simulink model "dvbs2_stream"  (R2024b)
settings: Solver=FixedStepDiscrete  StartTime=0.0  StopTime=18000/Fs  RelTol=1e-3
PreLoadFcn:
  | Rs = 125e3;
  | Fs = 8*Rs;
  | nsamp = 4096;
  | t = (0:nsamp)/Fs;
  | y = randi(2^8-1,1,2048);
  | ly = length(y);
InitFcn:
  | Rs = 125e3;
  | Fs = 8*Rs;
  | nsamp = 4096;
  | t = (0:nsamp)/Fs;
  | y = randi(2^8-1,1,2048);
  | ly = length(y);
libraries: hdlsllib x132, simulink x41, dspsigops x7, commseqgen3 x5, whdlutilities x5, commhdlcrc x2, dsphdlfiltering2 x1, whdlmod x1, sdrzblksprivate x1
(part 6 of 6)

== matlab function dvbs2_stream/HDL_DUT/Tx/DVB-S2 Tx/FEC Encoder/DVB-S2 LDPC Encoder/ParityController ==
  data: ird_addr output; pwr_addr output; pwr_enb output; prd_addr output; endEnc input; paraddr input; encenable input; inpLen input; parLen input; qfactor input; noofcol input; reset input; starto output; endo output; valido output; par_ind output; i_index output; p_index output; framevalid input
function [ird_addr,pwr_addr,pwr_enb,prd_addr,starto,endo,valido,par_ind,...
    i_index,p_index] = ParityController(endEnc,paraddr,encenable,...
    inpLen,parLen,qfactor,noofcol,reset,framevalid)

persistent validO prdAddr pwrAddr pwrEnb pwrEnbReg ...
    irdAddr prdEnb endValid startO icountZ inCount ...
    parCount pcountZ;
if isempty(validO)
    validO = false;
    prdAddr = uint8(1);
    pwrAddr = uint8(0);
    irdAddr = uint8(1);
    pwrEnb = false;
    pwrEnbReg = false;
    prdEnb = false;
    endValid = false;
    startO = false;
    icountZ = fi(1,0,9,0,hdlfimath);
    pcountZ = fi(1,0,9,0,hdlfimath);
    inCount = fi(0,0,16,0,hdlfimath);
    parCount = fi(0,0,16,0,hdlfimath);
end

ird_addr = irdAddr;
pwr_addr = pwrAddr;
prd_addr = prdAddr;
pwr_enb =  pwrEnbReg;
starto = startO;
par_ind = prdEnb;

i_index = icountZ;
p_index = pcountZ;

% Control signals
startO = endEnc;
endo = endValid;
valido = validO && ~endValid;

pwrEnbReg(:) = pwrEnb;

if reset
    prdAddr(:) = 1;
    pwrAddr(:) = 0;
    pwrEnb(:) = false;
    prdEnb(:) = false;
    endValid(:) = false;
    irdAddr(:) = 1;
    icountZ(:) = 1;
    pcountZ(:) = 1;
    inCount(:) = 0;
    parCount(:) = 0;
else
    if validO
        pwrEnb(:) = false;
        pwrAddr(:) = 0;

        if ~prdEnb
            if icountZ == fi(360,0,9,0,hdlfimath)
                if ~(irdAddr == noofcol)
                    irdAddr(:) = irdAddr + 1;
                end
                icountZ(:) = 1;
            else
                icountZ(:) = icountZ + 1;
            end
        end

        if inCount == inpLen
            prdEnb(:) = true;
        else
            inCount(:) = inCount + 1;
        end

        if prdEnb
            if parCount == parLen
                prdEnb(:) = false;
                endValid(:) = true;
            else
                parCount(:) = parCount + 1;
                if prdAddr == fi(qfactor,0,9,0,hdlfimath)
                    prdAddr(:) = 1;
                    if pcountZ == fi(360,0,9,0,hdlfimath)
                        pcountZ(:) = 1;
                    else
                        pcountZ(:) = pcountZ + 1;
                    end
                else
                    prdAddr(:) = prdAddr + 1;
                end
            end
        else
            prdAddr(:) = 1;
            endValid(:) = false;
        end
    else
        if framevalid
            pwrEnb(:) = true;
            if pwrAddr == uint8(255)
                pwrAddr(:) = 1;
            else
                pwrAddr(:) = pwrAddr+1;
            end
        else
            if encenable
                pwrEnb(:) = true;
            else
                pwrEnb(:) = false;
            end
            pwrAddr(:) = prdAddr;
        end
        prdAddr(:) = paraddr;
        prdEnb(:) = false;
        endValid(:) = false;
    end
end

if reset || endValid
    validO(:) = false;
elseif endEnc
    validO(:) = true;
end

== matlab function dvbs2_stream/HDL_DUT/Tx/DVB-S2 Tx/FEC Encoder/DVB-S2 LDPC Encoder/inputController ==
  data: reset output; datai input; iwr_data output size=360; iwr_addr output; starti input; endi input; validi input; fecframe input; coderate input; iwr_enb output size=360; ird_addr output; encenable output; addridx output; rdenable input; encend input; framevalid output; noofcol input
function [reset,iwr_data, iwr_addr,iwr_enb,ird_addr,encenable,addridx,framevalid] = ...
    inputController(datai,starti,endi,validi,fecframe,coderate,rdenable,encend,noofcol)
%#codegen

persistent fecFrame codeRate dataReg endReg validReg frameValid  frameValidReg...
           iwrData iwrAddr iwrEnb irdAddr idxCount wrCount encEnb disValid;
if isempty(dataReg)
    fecFrame = fi(0,0,1,0);
    codeRate = fi(0,0,4,0);
    dataReg = cast(0,'like',datai);
    endReg = false;
    validReg = false;
    frameValid = false;
    frameValidReg = false;
    iwrData = cast(zeros(360,1),'like',datai);
    iwrAddr = fi(0,0,8,0,hdlfimath);
    iwrEnb  = zeros(360,1)>0;
    irdAddr = fi(0,0,8,0,hdlfimath);
    idxCount = fi(1,0,9,0,hdlfimath);
    wrCount = fi(1,0,8,0,hdlfimath);
    encEnb = false;
    disValid = false;
end

% outputs
iwr_data = iwrData;
iwr_addr = iwrAddr;
iwr_enb = iwrEnb;
ird_addr = irdAddr;
encenable = disValid;

%% reset signal
reset = starti && validi;

%% Sample fecFrame and codeRate - Calculate input,parity length and address index.
if reset
    fecFrame(:) = fecframe;
    codeRate(:) = coderate;
end

addridx = fi(bitconcat(fecFrame,codeRate),0,5,0);

%% Reading data
if reset
    irdAddr(:) = 1;
else
    if rdenable
        if irdAddr == cast(noofcol,'like',irdAddr)
            irdAddr(:) = 1;
        else
            irdAddr(:) = irdAddr + 1;
        end
    end
end

%% Writing and Reading data into Input Bits RAM
if reset
    iwrData(:) = zeros(360,1);
    iwrAddr(:) = 0;
    iwrEnb(:) = zeros(360,1);
    idxCount(:) = 1;
    wrCount(:) = 1;
else
    if frameValid && validReg
        for idx = 1:360
            if idxCount == fi(idx,0,9,0)
                iwrEnb(idx) = true;
                iwrData(idx) = dataReg;
            else
                iwrEnb(idx) = false;
                iwrData(idx) = 0;
            end
        end
        iwrAddr(:) = wrCount;
        if idxCount == fi(360,0,9,0)
            idxCount(:) = 1;
            wrCount(:) = wrCount + 1;
        else
            idxCount(:) = idxCount + 1;
        end
    else
        iwrData(:) = 0;
        iwrEnb(:)  = false;
    end
end

if reset
    frameValid(:) = true;
    encEnb(:) = false;
elseif endReg && validReg
    frameValid(:) = false;
    encEnb(:) = true;
elseif encend
    encEnb(:) = false;
end

if reset
    frameValidReg(:) = true;
elseif endi && validi
    frameValidReg(:) = false;
end

if encEnb
    disValid(:) = ~disValid;
else
    disValid(:) = false;
end

framevalid = frameValidReg;

dataReg(:) = datai;
endReg(:) = endi;
validReg(:) = validi;

== matlab function dvbs2_stream/HDL_DUT/Tx/DVB-S2 Tx/Interleaver/DVB-S2 HDL Interleaver/RAM Address Generator/Read Offset Address/Read Offset Address Signals Generator/FIFO 3 Variables/No HDL/RAM status ==
  data: full output; ncount output; wr input; empty output; rd input
function [full,ncount,empty] = fcn(wr,rd)
%#codegen
     
    WL = 3;
    persistent count;
    if isempty(count)
        count = fi(0,0,WL+1,0,hdlfimath);
    end

    empty = (count == 0);
    full = (count > 2^WL-1);
    ncount = count;

    if wr
        count(:) = count + 1;
    end
    if rd
        count(:) = count - 1;
    end

end

== matlab function dvbs2_stream/Write Tx Data/Generate_Data ==
  data: TSorGS_Out output; DFL_Out output; UPL_Out output; SYNC_Out output; MODCOD_Out output; FECFRAME_Out output; nFrames parameter; nPackets parameter; TSorGS_In parameter; DFL_In parameter; UPL_In parameter; SYNC_In parameter; MODCOD_In parameter; FECFRAME_In parameter; frm_bits parameter; pkt_bits parameter; pl_cnt_bits parameter; frameEnd_pos parameter; frameStart_pos parameter; pktEnd_pos parameter; pktStart_pos parameter; data_Out output uint32
function [TSorGS_Out,DFL_Out,UPL_Out,SYNC_Out,MODCOD_Out,FECFRAME_Out, data_Out] = gendata_mask(nFrames,nPackets, ...
                                                                                                TSorGS_In,DFL_In,UPL_In,SYNC_In,MODCOD_In,FECFRAME_In, ...
                                                                                                frm_bits, pkt_bits, pl_cnt_bits, ...
                                                                                                frameEnd_pos, frameStart_pos, pktEnd_pos, pktStart_pos)

    
    [data_Out,TSorGS_Out,DFL_Out,UPL_Out,SYNC_Out,MODCOD_Out,FECFRAME_Out] = gendata(nFrames,nPackets, ...
                                                                                                TSorGS_In,DFL_In,UPL_In,SYNC_In,MODCOD_In,FECFRAME_In, ...
                                                                                                frm_bits, pkt_bits, pl_cnt_bits, ...
                                                                                                frameEnd_pos, frameStart_pos, pktEnd_pos, pktStart_pos);

end

== matlab function dvbs2_stream/HDL_DUT/Tx/MATLAB Function1 ==
  data: byteIn input; pktBitOut output; pktValidOut output; validIn input; readyOut output; LSBfirst input
% Serialise 8 bit number into 8 1 bit numbers
% On Valid In & Ready: Read dataIn
% next 8 cycles: dataIn bits are output on pktBitsOut
% If no valid input: Hold current output state
function [pktBitOut,pktValidOut,readyOut] = fcn(byteIn,validIn, LSBfirst)

    
    % Persistent Vars            
    persistent count;
    persistent byteInReg;
    if isempty(count)
        count = fi(1,0,log2(8)+1,0,hdlfimath);
        byteInReg = fi(0,0,8,0,hdlfimath);
    end

    % Other Vars
    it = fi(1,0,log2(8)+1,0,hdlfimath);

    % Extract bit

    if count == 1
        if validIn
            byteInReg(:) = byteIn;
            
            if LSBfirst
                it(:) = count;
            else
                it(:) = 8 - (count-1);
            end
            
            readyOut = false;
            pktValidOut = true;
            pktBitOut = bitget(byteInReg,it);
            count(:) = count + 1;
        else
            % Set Ready, wait for valid data
            count(:) = 1;
            it(:) = 1;
            readyOut = true;
            pktValidOut = false;
            pktBitOut = bitget(byteInReg,it);

        end
    elseif count < 8 && count > 1
        if LSBfirst
                it(:) = count;
            else
                it(:) = 8 - (count-1);
        end
        pktBitOut = bitget(byteInReg,it);
        pktValidOut = true;
        readyOut = false;
        count(:) = count + 1;            
    elseif count == 8
        if LSBfirst
                it(:) = count;
            else
                it(:) = 8 - (count-1);
        end
        pktBitOut = bitget(byteInReg,it);
        pktValidOut = true;
        readyOut = false;
        count(:) = 1;
    else
        count(:) = 1;
        it(:) = 1;
        readyOut = false;
        pktValidOut = false;
        pktBitOut = bitget(byteInReg,it);
    end
end

== matlab function dvbs2_stream/HDL_DUT/Tx/DVB-S2 Tx/BB Frame Generator/BB Header and Data CRC Generator/Data Field Generator/Packetized Streams/Discard SYNC ==
  data: dataIn input; dataOut output; startIn input; endIn input; validIn input; startOut output; endOut output; validOut output
function [dataOut,startOut,endOut,validOut] = discardSYNC(dataIn,startIn,endIn,validIn)
%#codegen


persistent count dataReg validReg startReg endReg;
    if isempty(count)
        count = fi(0,0,4,0,hdlfimath);
        dataReg = cast(0,'like',dataIn);
        validReg = false;
        startReg = false;
        endReg = false;
    end

    dataOut = dataReg;
    validOut = validReg;
    startOut = startReg;
    endOut = endReg;

    if startIn
        count(:) = 0;
    end
 
    if validIn
        if (count < 8)
            startReg = false;
            validReg = false;
        elseif count == 8
            startReg = true;
            validReg = true;
        else
            startReg = false;
            validReg = true;
        end
        if count < 9
            count(:) = count + 1;
        end
    else
        validReg = false;
        startReg = false;
    end
    if validReg
        dataReg = dataIn;
        endReg = endIn;
    else
        dataReg(:) = 0;
        endReg = false;
    end

end

== matlab function dvbs2_stream/HDL_DUT/Tx/DVB-S2 Tx/BB Frame Generator/BB Header and Data CRC Generator/Data Field Generator/Packetized Streams/MATLAB Function ==
  data: pktEndIn input; frameEndOut output; frameEndIn input
function frameEndOut = fcn(pktEndIn,frameEndIn)
%#codegen

    persistent frameEnded;
    if isempty(frameEnded)
        frameEnded = false;
    end

    if frameEndIn
        frameEnded = true;
    end

    if pktEndIn && frameEnded
        frameEndOut = true;
        frameEnded = false;
    else
        frameEndOut = false;
    end


end

== matlab function dvbs2_stream/HDL_DUT/Tx/DVB-S2 Tx/BB Frame Generator/BB Header and Data CRC Generator/MATLAB Function ==
  data: validIn input; startIn input; endIn input; validAppend output; DFL input; endAppend output
function [validAppend,endAppend] = DFLLengthCounter(validIn,startIn,endIn,DFL)
%#codegen
   
   MAX_DFL = 58192-80; 
   persistent countDFL isEndReceived;
   if isempty(countDFL)
       countDFL = fi(0,0,nextpow2(MAX_DFL),0,hdlfimath);
       isEndReceived = false;
   end
   
   if startIn
       countDFL(:) = 0;
   end

   if isEndReceived
       validAppend = true;
       countDFL(:) = countDFL + 1;
   elseif validIn
       validAppend = false;
       countDFL(:) = countDFL + 1;
   else
       validAppend = false;
   end
   
   if countDFL > DFL
       validAppend = false;
   end
   if DFL ~= 0
       if countDFL >= DFL
           endAppend = isEndReceived;
           isEndReceived = false;
       else
           endAppend = false;
       end
   else
       endAppend = false;
   end

   if endIn
       isEndReceived = true;
   end
end

== matlab function dvbs2_stream/HDL_DUT/Tx/DVB-S2 Tx/BB Frame Generator/BB Header and Data CRC Generator/No HDL/MATLAB Function1 ==
  data: u input; y output
function y = monostable(u)
%#codegen

   persistent count countActive;
   if isempty(count)
       count = fi(0,0,nextpow2(80),0,hdlfimath);
       countActive = false;
   end

   y = countActive;
    
   if count == 79
       countActive = false;
       count(:) = 0;
   end
   if countActive
       count(:) = count + 1;
   end
   if u 
       countActive = true;
   end

end

== matlab function dvbs2_stream/HDL_DUT/Tx/DVB-S2 Tx/BB Frame Generator/Data Store FIFO/MATLAB Function ==
  data: wr input; startIn input; validOut output; DFL input; endOut output
function [validOut,endOut] = DFLLengthCounter(wr,startIn,DFL)
%#codegen
   
   WL = 7;
   persistent countDFL countActive countSamplesInRAM;
   if isempty(countDFL)
       countDFL = cast(0,'like',DFL);
       countActive = false;
       countSamplesInRAM = fi(0,0,WL+1,0,hdlfimath);

   end

   empty = (countSamplesInRAM == 0);
   enb = ~empty;
   % cntActive = countActive;
   % cnt = countDFL;

   validOut = countActive && enb;
   endOut = countActive && (countDFL == DFL);


   if (DFL ~= 0) && (countDFL == DFL) && enb
       countActive = false;
   end

   if startIn
       countDFL(:) = 0;
       countActive = true;
   end

   if countActive && enb
       countDFL(:) = countDFL + 1;
   end



   if wr
       countSamplesInRAM(:) = countSamplesInRAM + 1;
   end
   if validOut % rd
       countSamplesInRAM(:) = countSamplesInRAM - 1;
   end



end

== matlab function dvbs2_stream/HDL_DUT/Tx/DVB-S2 Tx/BB Frame Generator/Data Store FIFO/No HDL/RAM status ==
  data: full output; ncount output; wr input; empty output; rd input
function [full,ncount,empty] = fcn(wr,rd)
%#codegen
     
    WL = 7;
    persistent count;
    if isempty(count)
        count = fi(0,0,WL+1,0,hdlfimath);
    end

    empty = (count == 0);
    full = (count > 2^WL-1);
    ncount = count;

    if wr
        count(:) = count + 1;
    end
    if rd
        count(:) = count - 1;
    end

end
